simulink model "Experimento3"  (R2023a)
settings: Solver=ode4  StartTime=0.0  StopTime=10.0  FixedStep=0.01  RelTol=1e-3
undefined symbols (not defined in the file): A, B, C, D, d1, G1, G2, G3, G4, G5, n1
settings Model: Creator=carlo  LastModifiedBy=carlo

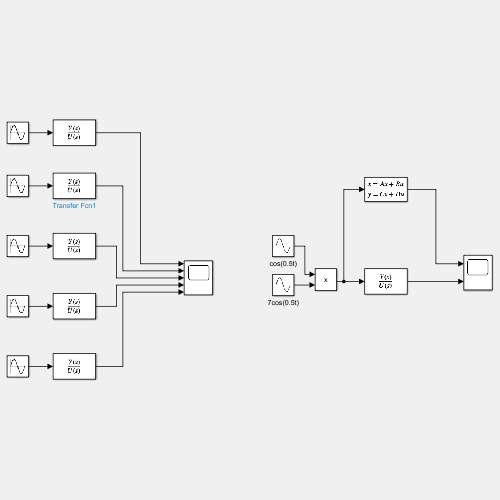
[thumbnail: Simulink's stored preview of the top-level diagram]
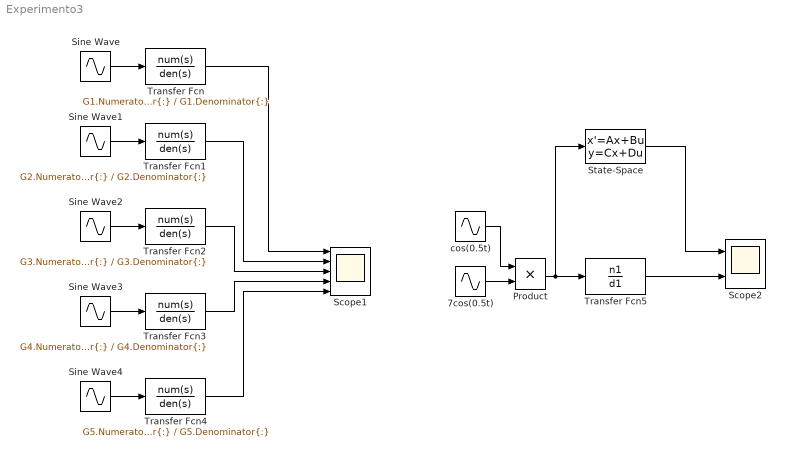
== system Experimento3 ==
  7cos(0.5t) : Sin  Amplitude=7  Frequency=0.5  Phase=90  SampleTime=0
  Product : Product
  Scope1 : Scope  NumInputPorts=5
  Scope2 : Scope  NumInputPorts=2
  Sine Wave{,1..4} (5 alike) : Sin  Frequency=2  SampleTime=0
  State-Space : StateSpace  A=A  B=B  C=C  D=D  InitialCondition=[0;0;0]
  Transfer Fcn : TransferFcn  Numerator=G1.Numerator{:}  Denominator=G1.Denominator{:}
  Transfer Fcn1 : TransferFcn  Numerator=G2.Numerator{:}  Denominator=G2.Denominator{:}
  Transfer Fcn2 : TransferFcn  Numerator=G3.Numerator{:}  Denominator=G3.Denominator{:}
  Transfer Fcn3 : TransferFcn  Numerator=G4.Numerator{:}  Denominator=G4.Denominator{:}
  Transfer Fcn4 : TransferFcn  Numerator=G5.Numerator{:}  Denominator=G5.Denominator{:}
  Transfer Fcn5 : TransferFcn  Numerator=n1  Denominator=d1
  cos(0.5t) : Sin  Frequency=0.5  Phase=90  SampleTime=0
  wires:
  Sine Wave/1 -> Transfer Fcn/1
  Sine Wave1/1 -> Transfer Fcn1/1
  Sine Wave2/1 -> Transfer Fcn2/1
  Sine Wave3/1 -> Transfer Fcn3/1
  Sine Wave4/1 -> Transfer Fcn4/1
  Transfer Fcn/1 -> Scope1/1
  Transfer Fcn1/1 -> Scope1/2
  Transfer Fcn2/1 -> Scope1/3
  Transfer Fcn3/1 -> Scope1/4
  Transfer Fcn4/1 -> Scope1/5
  cos(0.5t)/1 -> Product/1
  7cos(0.5t)/1 -> Product/2
  Product/1 -> State-Space/1, Transfer Fcn5/1
  Transfer Fcn5/1 -> Scope2/2
  State-Space/1 -> Scope2/1
